simulink model "open_diff"  (R2019b)
settings: Solver=VariableStepAuto  StartTime=0.0  StopTime=10.0  RelTol=1e-3
InitFcn:
  | J_1=0.1;
  | J_2=0.2;
  | T_d=1;
  | b_d=0.01;
  | J_d=0.1;
  | N=3;
  | eta=0.7;
  | b_1=0.01;
  | b_2=0.02;
settings Model: Creator=srikesh  LastModifiedBy=srikesh

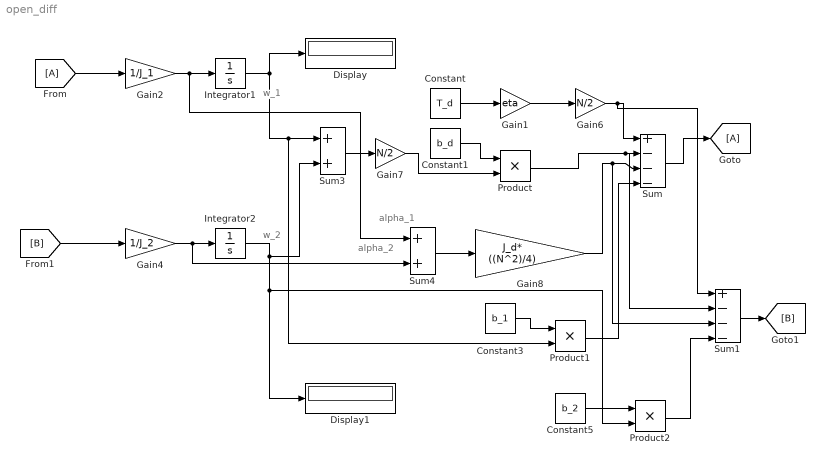
== system open_diff ==
  note: alpha_2
  note: alpha_1
  note: w_2
  note: w_1
  Constant : Constant  Value=T_d
  Constant1 : Constant  Value=b_d
  Constant3 : Constant  Value=b_1
  Constant5 : Constant  Value=b_2
  Display : Display
  Display1 : Display
  Gain1 : Gain  Gain=eta
  Gain2 : Gain  Gain=1/J_1
  Gain4 : Gain  Gain=1/J_2
  Gain6 : Gain  Gain=N/2
  Gain7 : Gain  Gain=N/2
  Gain8 : Gain  Gain=J_d* ((N^2)/4)
  Integrator1 : Integrator
  Integrator2 : Integrator
  Product : Product
  Product1 : Product
  Product2 : Product
  Sum : Sum  Inputs=+---
  Sum1 : Sum  Inputs=+---
  Sum3 : Sum
  Sum4 : Sum
  wires:
  Constant/1 -> Gain1/1
  Sum/1 -> [A]
  Constant1/1 -> Product/1
  Product/1 -> Sum1/2, Sum/2
  Integrator1/1 -> Sum3/1, Product1/2, Display/1
  Constant3/1 -> Product1/1
  Gain2/1 -> Sum4/1, Integrator1/1
  [A] -> Gain2/1
  [B] -> Gain4/1
  Gain4/1 -> Sum4/2, Integrator2/1
  Constant5/1 -> Product2/1
  Integrator2/1 -> Sum3/2, Display1/1, Product2/2
  Gain1/1 -> Gain6/1
  Gain6/1 -> Sum1/1, Sum/1
  Sum3/1 -> Gain7/1
  Gain7/1 -> Product/2
  Sum4/1 -> Gain8/1
  Gain8/1 -> Sum1/3, Sum/3
  Product1/1 -> Sum/4
  Product2/1 -> Sum1/4
  Sum1/1 -> [B]
